simulink model "transform"  (R2018b)
settings: Solver=VariableStepAuto  StartTime=0.0  StopTime=10.0  RelTol=1e-3
settings Model: Creator=frodan  LastModifiedBy=frodan

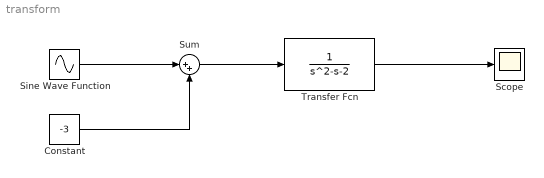
== system transform ==
  Constant : Constant  Value=-3
  Scope : Scope
  Sine Wave Function : Sin  Frequency=2  SampleTime=0
  Sum : Sum  Inputs=|++
  Transfer Fcn : TransferFcn  Denominator=[1 -1 -2]
  wires:
  Transfer Fcn/1 -> Scope/1
  Sum/1 -> Transfer Fcn/1
  Constant/1 -> Sum/2
  Sine Wave Function/1 -> Sum/1
